simulink model "HLR_10a"  (R2024a)
settings: configuration reference "mdlCheck_config_allPass_codeGen" (kept outside this file)
settings Model: DataDictionary=ModeLogic_data.sldd  Creator=manthony  LastModifiedBy=dlheureu
settings ConfigSetRef: SourceName=mdlCheck_config_allPass_codeGen

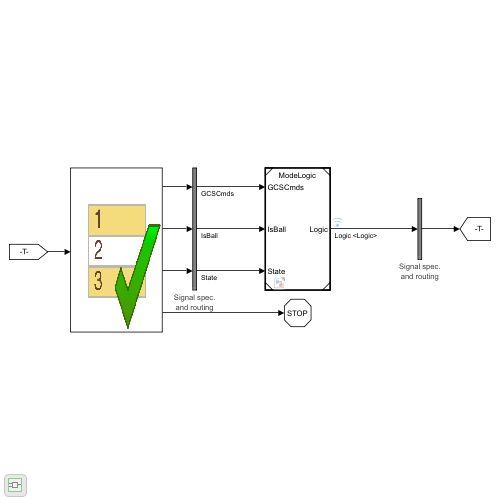
[thumbnail: Simulink's stored preview of the top-level diagram]
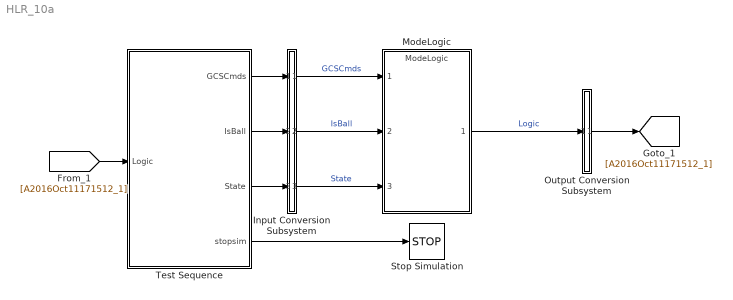
== system HLR_10a ==
  Input Conversion Subsystem : Subsystem  Tag=__SLT_ICS__  Description=|
      | Signal spec.
      | and routing
      settings: AttributesFormatString=%<Description>
  ModeLogic : ModelReference  ModelNameDialog=ModeLogic  SimulationMode=Normal  ModelReferenceVersion=2.10
  Output Conversion Subsystem : Subsystem  Tag=__SLT_OCS__  Description=|
      | Signal spec.
      | and routing
      mask init:
      | ICDictionary = get_param(bdroot, 'DataDictionary');
      | if isempty(ICDictionary)
      |    ICScope = Simulink.data.BaseWorkspace;
      | else
      |    ICScope = Simulink.data.DataDictionary(ICDictionary);
      | end
      | 
      | IC1 = Simulink.Bus.createMATLABStruct('Logic', [], [1 1], ICScope);
      settings: AttributesFormatString=%<Description>
  Stop Simulation : Stop
  Test Sequence : Test Sequence  TreatAsAtomicUnit=on
  wires:
  [A2016Oct11171512_1] -> Test Sequence/1(Logic)
  Test Sequence/4(stopsim) -> Stop Simulation/1
  Test Sequence/1(GCSCmds) -> Input Conversion Subsystem/1(Inport_1)
  Test Sequence/2(IsBall) -> Input Conversion Subsystem/2(Inport_2)
  Test Sequence/3(State) -> Input Conversion Subsystem/3(Inport_3)
  Output Conversion Subsystem/1(Outport_1) -> [A2016Oct11171512_1]
  ModeLogic/1 -> Output Conversion Subsystem/1(Inport_1)  "Logic"
  Input Conversion Subsystem/1(Outport_1) -> ModeLogic/1  "GCSCmds"
  Input Conversion Subsystem/2(Outport_2) -> ModeLogic/2  "IsBall"
  Input Conversion Subsystem/3(Outport_3) -> ModeLogic/3  "State"

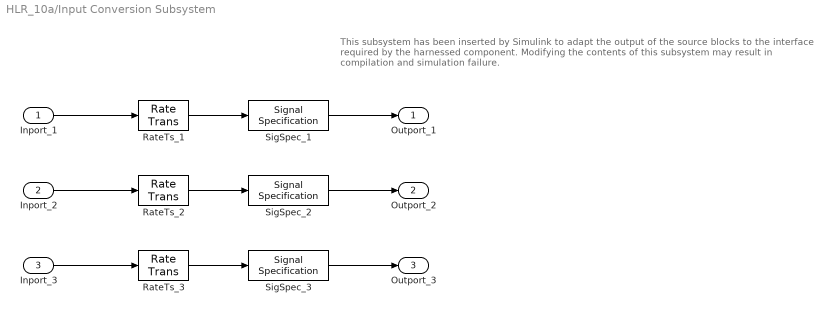
== system HLR_10a/Input Conversion Subsystem ==
  note: This subsystem has been inserted by Simulink to adapt the output of the source blocks to the interface required by the harnessed component.
      |  Modifying the contents of this subsystem may result in compilation and simulation failure.
  Inport_1 : Inport
  Inport_2 : Inport  Port=2
  Inport_3 : Inport  Port=3
  RateTs_1 : RateTransition  OutPortSampleTime=0.1
  RateTs_2 : RateTransition  OutPortSampleTime=0.1
  RateTs_3 : RateTransition  OutPortSampleTime=0.1
  SigSpec_1 : SignalSpecification  OutDataTypeStr=Bus: GCSCommands  Dimensions=[1]  SampleTime=0.1  BusOutputAsStruct=on
  SigSpec_2 : SignalSpecification  OutDataTypeStr=boolean  Dimensions=[1]  SampleTime=0.1
  SigSpec_3 : SignalSpecification  OutDataTypeStr=Bus: State  Dimensions=[1]  SampleTime=0.1  BusOutputAsStruct=on
  Outport_1 : Outport
  Outport_2 : Outport  Port=2
  Outport_3 : Outport  Port=3
  wires:
  SigSpec_1/1 -> Outport_1/1
  RateTs_1/1 -> SigSpec_1/1
  Inport_1/1 -> RateTs_1/1
  SigSpec_2/1 -> Outport_2/1
  RateTs_2/1 -> SigSpec_2/1
  Inport_2/1 -> RateTs_2/1
  SigSpec_3/1 -> Outport_3/1
  RateTs_3/1 -> SigSpec_3/1
  Inport_3/1 -> RateTs_3/1

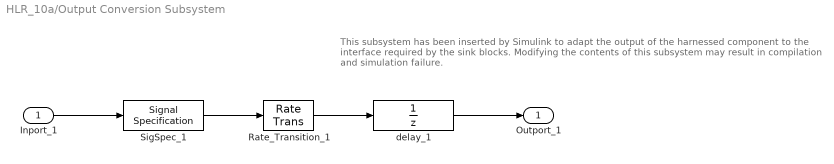
== system HLR_10a/Output Conversion Subsystem ==
  note: This subsystem has been inserted by Simulink to adapt the output of the harnessed component to the interface required by the sink blocks.
      |  Modifying the contents of this subsystem may result in compilation and simulation failure.
  Inport_1 : Inport
  Rate_Transition_1 : RateTransition  OutPortSampleTimeOpt=Inherit
  SigSpec_1 : SignalSpecification  OutDataTypeStr=Bus: Logic  Dimensions=[1]  SampleTime=0.1  BusOutputAsStruct=on
  delay_1 : UnitDelay  InitialCondition=IC1  SampleTime=-1
  Outport_1 : Outport
  wires:
  Inport_1/1 -> SigSpec_1/1
  SigSpec_1/1 -> Rate_Transition_1/1
  Rate_Transition_1/1 -> delay_1/1
  delay_1/1 -> Outport_1/1

== stateflow chart HLR_10a/Test Sequence ==
  state Init
    %% Initialize data outputs.
    GCSCmds.EMERGENCY_OFF = false;
    GCSCmds.WIFIconnected = false;
    GCSCmds.BTconnected = false;
    GCSCmds.CalibrateCmd = false;
    GCSCmds.GCS_MissionMode = uint8(0);
    GCSCmds.GCS_HeadingCmd = single(0);
    IsBall = false;
    State.CalibrationDone = false;
    State.Pos_BODY = single(zeros(3, 1));
    State.Pos_FSD = single(zeros(3, 1));
    State.V_BODY = single(zeros(3, 1));
    State.V_FSD = single(zeros(3, 1));
    State.Acc_BODY = single(zeros(3, 1));
    State.Acc_FSD = single(zeros(3, 1));
    State.AngRate = single(zeros(3, 1));
    State.Angles = single(zeros(3, 1));
    State.Heading = single(0);
    State.Altitude = single(0);
    State.BatteryVolts = single(3.3);
    settings: description=Initialize all inputs
  state Wifi_and_BT_on
    GCSCmds.WIFIconnected = true;
    GCSCmds.BTconnected = true;
  state Calibration
    GCSCmds.CalibrateCmd = true;
  state CalibrationDone
    State.CalibrationDone = true;
    GCSCmds.GCS_MissionMode = uint8(1);
  state SeeBall
    IsBall = true;
  state Wait
    verify( Logic.Mode == uint8(5) );
  state Crash_Commanded
    %From TrackAlt
    verify( Logic.Mode == uint8(5) );
    GCSCmds.EMERGENCY_OFF = true;
  state Verify
    verify( Logic.Mode == uint8(9) );
    stopsim = true;
  (default) -> Init
  Init -> Wifi_and_BT_on : [
      | after(1,tick)
      | ]
  Wifi_and_BT_on -> Calibration : [
      | after(1,tick)
      | ]
  Calibration -> CalibrationDone : [
      | after(1,tick)
      | ]
  CalibrationDone -> SeeBall : [
      | after(1,tick)
      | ]
  SeeBall -> Wait : [
      | after(1,tick)
      | ]
  Wait -> Crash_Commanded : [
      | after(1,tick)
      | ]
  Crash_Commanded -> Verify : [after(1,tick)
      | ]
  data: Logic input Bus: Logic size=[1]; GCSCmds output Bus: GCSCommands size=[1] =0; IsBall output boolean size=[1]; State output Bus: State size=[1] =0; stopsim output boolean =false
